simulink model "Slip_ratio"  (R2023b)
settings: Solver=ode5  StartTime=0.0  StopTime=10.0  FixedStep=0.001  RelTol=1e-3
settings Model: Creator=ibaad  LastModifiedBy=ajame

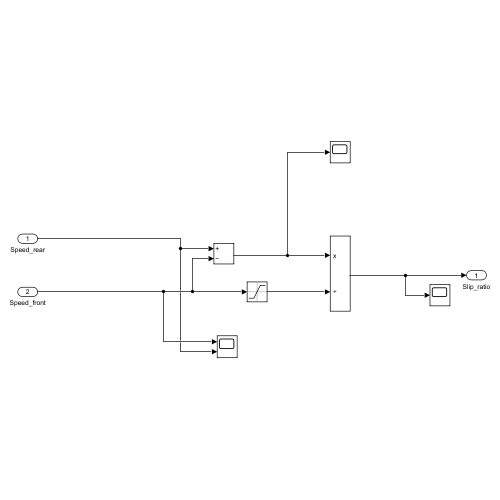
[thumbnail: Simulink's stored preview of the top-level diagram]
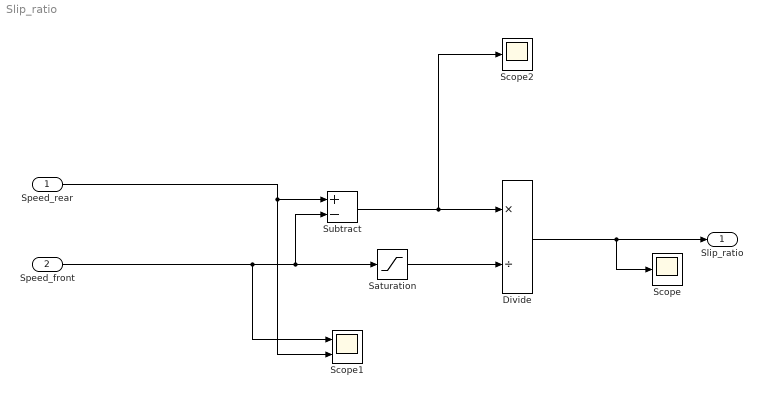
== system Slip_ratio ==
  Speed_rear : Inport
  Speed_front : Inport  Port=2
  Divide : Product  Inputs=*/  RndMeth=Round
  Saturation : Saturate  UpperLimit=200  LowerLimit=0.1
  Scope : Scope
  Scope1 : Scope  NumInputPorts=2
  Scope2 : Scope
  Subtract : Sum  Inputs=+-
  Slip_ratio : Outport
  wires:
  Speed_rear/1 -> Scope1/2, Subtract/1
  Speed_front/1 -> Scope1/1, Saturation/1, Subtract/2
  Subtract/1 -> Scope2/1, Divide/1
  Divide/1 -> Scope/1, Slip_ratio/1
  Saturation/1 -> Divide/2
